simulink model "test_TankSensing2"  (R2022b)
settings: Solver=FixedStepDiscrete  StartTime=0.0  StopTime=10.0  FixedStep=0.0001  RelTol=1e-3
undefined symbols (not defined in the file or in its folder): hil_TankSensing_lib, ResToGnd, ResToVcc, tanksensing_lib, Vcc
libraries: simulink x4
settings Model: Creator=CentoPas  LastModifiedBy=Km
settings SolverCC: AlgebraicLoopSolver=TrustRegion
settings DebuggingCC: UnconnectedInputMsg=warning  UnconnectedOutputMsg=warning  UnconnectedLineMsg=warning  SFMachineParentedDataDiag=warning
settings ModelReferenceCC: EnableRefExpFcnMdlSchedulingChecks=on

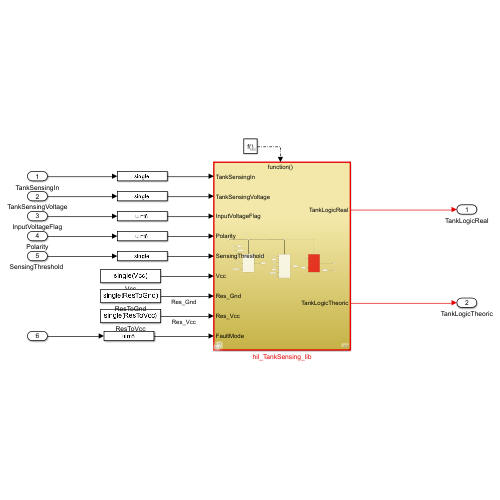
[thumbnail: Simulink's stored preview of the top-level diagram]
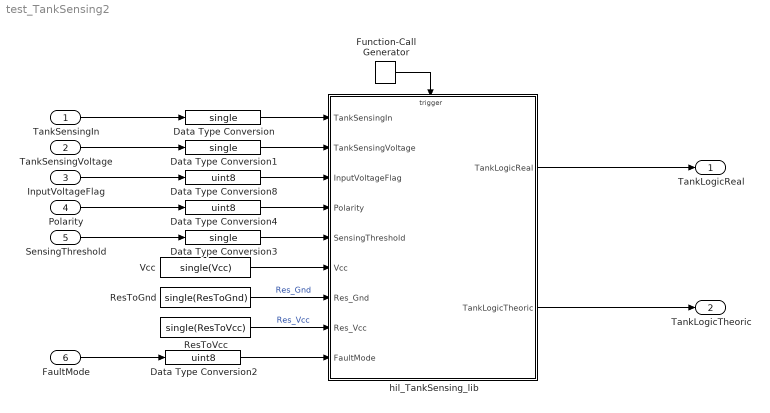
== system test_TankSensing2 ==
  TankSensingIn : Inport  OutDataTypeStr=single
  TankSensingVoltage : Inport  Port=2  OutDataTypeStr=single
  InputVoltageFlag : Inport  Port=3  OutDataTypeStr=uint8
  Polarity : Inport  Port=4  OutDataTypeStr=uint8
  "SensingThreshold " : Inport  Port=5  OutDataTypeStr=single
  FaultMode : Inport  Port=6  OutDataTypeStr=uint8
  Data Type Conversion : DataTypeConversion  OutDataTypeStr=single  SaturateOnIntegerOverflow=off  RndMeth=Floor
  Data Type Conversion1 : DataTypeConversion  OutDataTypeStr=single  SaturateOnIntegerOverflow=off  RndMeth=Floor
  Data Type Conversion2 : DataTypeConversion  OutDataTypeStr=uint8  SaturateOnIntegerOverflow=off  RndMeth=Floor
  Data Type Conversion3 : DataTypeConversion  OutDataTypeStr=single  SaturateOnIntegerOverflow=off  RndMeth=Floor
  Data Type Conversion4 : DataTypeConversion  OutDataTypeStr=uint8  SaturateOnIntegerOverflow=off  RndMeth=Floor
  Data Type Conversion8 : DataTypeConversion  OutDataTypeStr=uint8  SaturateOnIntegerOverflow=off  RndMeth=Floor
  Function-Call Generator : simulink/Ports & Subsystems/Function-Call Generator  sample_time=0.001  numberOfIterations=1  DisallowWideOutput=off
  ResToGnd : Constant  Value=single(ResToGnd)
  ResToVcc : Constant  Value=single(ResToVcc)
  Vcc : Constant  Value=single(Vcc)  OutDataTypeStr=single
  hil_TankSensing_lib : Subsystem  AncestorBlock=tanksensing_lib/hil_TankSensing_lib  TreatAsAtomicUnit=on  RTWFcnName=hil_tanksensing_lib
      settings: LibrarySourceBlock=tanksensing_lib/hil_TankSensing_lib  RTWFcnNameOpts=User specified
  TankLogicReal : Outport  OutDataTypeStr=uint8
  TankLogicTheoric : Outport  Port=2  OutDataTypeStr=uint8
  wires:
  Function-Call Generator/1 -> hil_TankSensing_lib/Trigger
  hil_TankSensing_lib/1(TankLogicReal) -> TankLogicReal/1
  hil_TankSensing_lib/2(TankLogicTheoric) -> TankLogicTheoric/1
  Data Type Conversion4/1 -> hil_TankSensing_lib/4(Polarity)
  Data Type Conversion3/1 -> hil_TankSensing_lib/5("SensingThreshold ")
  Vcc/1 -> hil_TankSensing_lib/6(Vcc)
  FaultMode/1 -> Data Type Conversion2/1
  ResToVcc/1 -> hil_TankSensing_lib/8(Res_Vcc)  "Res_Vcc"
  Data Type Conversion1/1 -> hil_TankSensing_lib/2(TankSensingVoltage)
  Data Type Conversion/1 -> hil_TankSensing_lib/1(TankSensingIn)
  Data Type Conversion8/1 -> hil_TankSensing_lib/3(InputVoltageFlag)
  ResToGnd/1 -> hil_TankSensing_lib/7(Res_Gnd)  "Res_Gnd"
  TankSensingIn/1 -> Data Type Conversion/1
  TankSensingVoltage/1 -> Data Type Conversion1/1
  InputVoltageFlag/1 -> Data Type Conversion8/1
  Polarity/1 -> Data Type Conversion4/1
  "SensingThreshold "/1 -> Data Type Conversion3/1
  Data Type Conversion2/1 -> hil_TankSensing_lib/9("FaultMode ")

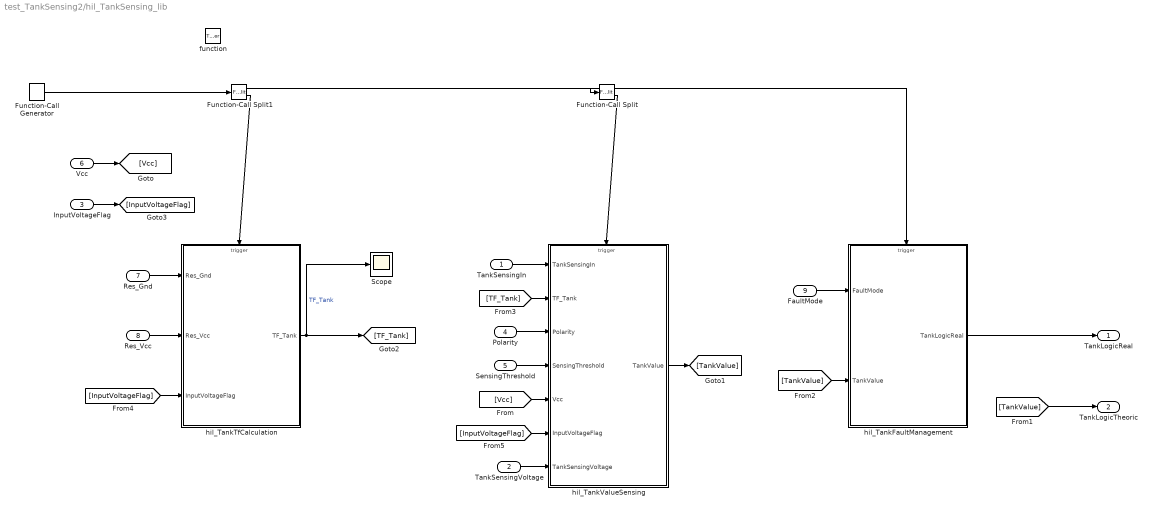
== system test_TankSensing2/hil_TankSensing_lib ==
  TankSensingIn : Inport  RequirementInfo={} %GIDa_b751ddf4_f7ab_455b_ad5f_57267e982822
  TankSensingVoltage : Inport  Port=2
  InputVoltageFlag : Inport  Port=3
  Polarity : Inport  Port=4
  "SensingThreshold " : Inport  Port=5
  Vcc : Inport  RequirementInfo={} %GIDa_577f5463_3c1c_4139_8bd3_238316ee9637  Port=6
  Res_Gnd : Inport  Port=7
  Res_Vcc : Inport  Port=8
  "FaultMode " : Inport  Port=9
  function : TriggerPort  TriggerType=function-call  VariantControl=Variant
  Function-Call Generator : simulink/Ports & Subsystems/Function-Call Generator  sample_time=-1  numberOfIterations=1  DisallowWideOutput=off
  Function-Call Split : FunctionCallSplit  NumOutputPorts=2  OutputPortLayout=default
  Function-Call Split1 : FunctionCallSplit  NumOutputPorts=2  OutputPortLayout=default
  Scope : Scope
  hil_TankFaultManagement : Subsystem  TreatAsAtomicUnit=on
  hil_TankTfCalculation : Subsystem  TreatAsAtomicUnit=on
  hil_TankValueSensing : Subsystem  TreatAsAtomicUnit=on
  TankLogicReal : Outport  OutDataTypeStr=uint8
  TankLogicTheoric : Outport  Port=2  OutDataTypeStr=uint8
  wires:
  TankSensingVoltage/1 -> hil_TankValueSensing/7(TankSensingVoltage)
  [InputVoltageFlag] -> hil_TankValueSensing/6(InputVoltageFlag)
  [InputVoltageFlag] -> hil_TankTfCalculation/3(InputVoltageFlag)
  InputVoltageFlag/1 -> [InputVoltageFlag]
  Res_Vcc/1 -> hil_TankTfCalculation/2(Res_Vcc)
  Res_Gnd/1 -> hil_TankTfCalculation/1(Res_Gnd)
  hil_TankTfCalculation/1(TF_Tank) -> Scope/1, [TF_Tank]  "TF_Tank"
  Function-Call Split1/2 -> hil_TankTfCalculation/Trigger
  Function-Call Split1/1 -> Function-Call Split/1
  Function-Call Generator/1 -> Function-Call Split1/1
  [TankValue] -> TankLogicTheoric/1
  hil_TankFaultManagement/1(TankLogicReal) -> TankLogicReal/1
  "FaultMode "/1 -> hil_TankFaultManagement/1(FaultMode)
  [TankValue] -> hil_TankFaultManagement/2(TankValue)
  [Vcc] -> hil_TankValueSensing/5("Vcc ")
  "SensingThreshold "/1 -> hil_TankValueSensing/4(SensingThreshold)
  Polarity/1 -> hil_TankValueSensing/3(Polarity)
  [TF_Tank] -> hil_TankValueSensing/2(TF_Tank)
  hil_TankValueSensing/1("TankValue ") -> [TankValue]
  Function-Call Split/1 -> hil_TankFaultManagement/Trigger
  Vcc/1 -> [Vcc]
  Function-Call Split/2 -> hil_TankValueSensing/Trigger
  TankSensingIn/1 -> hil_TankValueSensing/1(TankSensingIn)

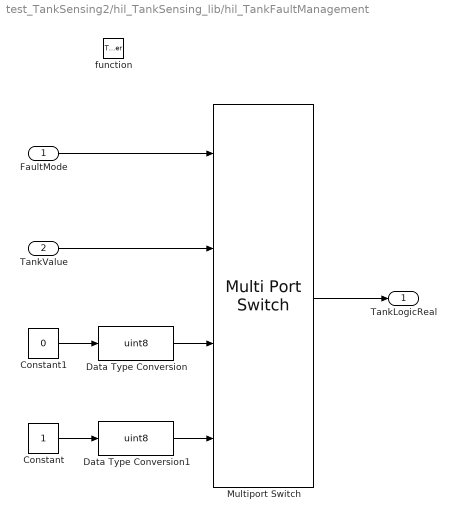
== system test_TankSensing2/hil_TankSensing_lib/hil_TankFaultManagement ==
  FaultMode : Inport
  TankValue : Inport  Port=2
  function : TriggerPort  TriggerType=function-call  VariantControl=Variant
  Constant : Constant
  Constant1 : Constant  Value=0
  Data Type Conversion : DataTypeConversion  OutDataTypeStr=uint8  SaturateOnIntegerOverflow=off  RndMeth=Floor
  Data Type Conversion1 : DataTypeConversion  OutDataTypeStr=uint8  SaturateOnIntegerOverflow=off  RndMeth=Floor
  Multiport Switch : MultiPortSwitch  DataPortOrder=Zero-based contiguous  zeroidx=on  SaturateOnIntegerOverflow=off  InputSameDT=off
  TankLogicReal : Outport
  wires:
  Data Type Conversion1/1 -> Multiport Switch/4
  Data Type Conversion/1 -> Multiport Switch/3
  Constant/1 -> Data Type Conversion1/1
  Constant1/1 -> Data Type Conversion/1
  TankValue/1 -> Multiport Switch/2
  FaultMode/1 -> Multiport Switch/1
  Multiport Switch/1 -> TankLogicReal/1

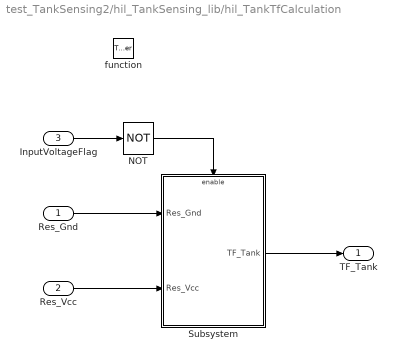
== system test_TankSensing2/hil_TankSensing_lib/hil_TankTfCalculation ==
  Res_Gnd : Inport
  Res_Vcc : Inport  Port=2
  InputVoltageFlag : Inport  Port=3
  function : TriggerPort  TriggerType=function-call  VariantControl=Variant
  NOT : Logic  Operator=NOT  IconShape=distinctive  AllPortsSameDT=off  OutDataTypeStr=boolean
  Subsystem : Subsystem
  TF_Tank : Outport  OutDataTypeStr=single
  wires:
  NOT/1 -> Subsystem/Enable
  InputVoltageFlag/1 -> NOT/1
  Subsystem/1(TF_Tank) -> TF_Tank/1
  Res_Vcc/1 -> Subsystem/2(Res_Vcc)
  Res_Gnd/1 -> Subsystem/1(Res_Gnd)

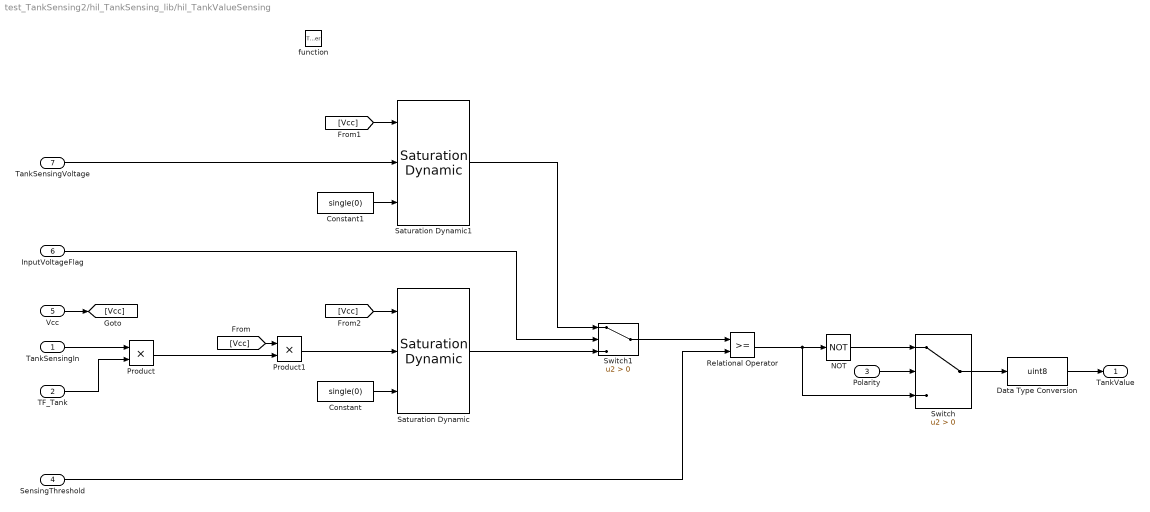
== system test_TankSensing2/hil_TankSensing_lib/hil_TankValueSensing ==
  TankSensingIn : Inport
  TF_Tank : Inport  Port=2
  Polarity : Inport  Port=3
  SensingThreshold : Inport  Port=4
  "Vcc " : Inport  Port=5
  InputVoltageFlag : Inport  Port=6
  TankSensingVoltage : Inport  Port=7
  function : TriggerPort  TriggerType=function-call  VariantControl=Variant
  Constant : Constant  Value=single(0)
  Constant1 : Constant  Value=single(0)
  Data Type Conversion : DataTypeConversion  OutDataTypeStr=uint8  SaturateOnIntegerOverflow=off  RndMeth=Floor
  NOT : Logic  Operator=NOT  IconShape=distinctive  AllPortsSameDT=off  OutDataTypeStr=boolean
  Product : Product
  Product1 : Product
  Relational Operator : RelationalOperator  OutDataTypeStr=boolean  RndMeth=Zero  InputSameDT=off
  Saturation Dynamic : simulink/Discontinuities/Saturation Dynamic  OutMin=[]  OutMax=[]  OutDataTypeStr=Inherit: Same as second input  OutDataType=fixdt(1, 16)  OutScaling=2^-10  DoSatur=off
  Saturation Dynamic1 : simulink/Discontinuities/Saturation Dynamic  OutMin=[]  OutMax=[]  OutDataTypeStr=Inherit: Same as second input  OutDataType=fixdt(1, 16)  OutScaling=2^-10  DoSatur=off
  Switch : Switch  Criteria=u2 > Threshold  SaturateOnIntegerOverflow=off  InputSameDT=off
  Switch1 : Switch  Criteria=u2 > Threshold  SaturateOnIntegerOverflow=off  InputSameDT=off
  "TankValue " : Outport
  wires:
  [Vcc] -> Saturation Dynamic/1
  [Vcc] -> Saturation Dynamic1/1
  [Vcc] -> Product1/1
  "Vcc "/1 -> [Vcc]
  Constant1/1 -> Saturation Dynamic1/3
  Saturation Dynamic1/1 -> Switch1/1
  TankSensingVoltage/1 -> Saturation Dynamic1/2
  Saturation Dynamic/1 -> Switch1/3
  InputVoltageFlag/1 -> Switch1/2
  Switch1/1 -> Relational Operator/1
  Product1/1 -> Saturation Dynamic/2
  Product/1 -> Product1/2
  Data Type Conversion/1 -> "TankValue "/1
  Relational Operator/1 -> NOT/1, Switch/3
  Constant/1 -> Saturation Dynamic/3
  NOT/1 -> Switch/1
  Switch/1 -> Data Type Conversion/1
  Polarity/1 -> Switch/2
  TankSensingIn/1 -> Product/1
  SensingThreshold/1 -> Relational Operator/2
  TF_Tank/1 -> Product/2

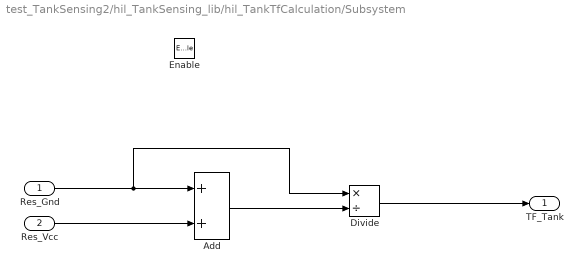
== system test_TankSensing2/hil_TankSensing_lib/hil_TankTfCalculation/Subsystem ==
  Res_Gnd : Inport
  Res_Vcc : Inport  Port=2
  Enable : EnablePort
  Add : Sum
  Divide : Product  Inputs=*/
  TF_Tank : Outport  OutDataTypeStr=single
  wires:
  Res_Gnd/1 -> Add/1, Divide/1
  Res_Vcc/1 -> Add/2
  Divide/1 -> TF_Tank/1
  Add/1 -> Divide/2
